simulink model "tracking_model"  (R2017a)
settings: Solver=VariableStepAuto  StartTime=0.0  StopTime=10.0  RelTol=1e-3
values from neighbouring files (symbols this model uses):
  x0 = 100    [validate_model.m]
undefined symbols (not defined in the file or in its folder): sys
(part 14 of 14)

== matlab function tracking_model/Plant/Dynamic system/Mass_block/mass_tensor ==
  data: in1 input; M_matrix output
function M_matrix = Mass_matrix(in1)

%    This function was generated by the Symbolic Math Toolbox version 7.2.

%    10-Jan-2021 16:43:29



th = in1(3,:);

th1 = in1(4,:);

th2 = in1(5,:);

th3 = in1(6,:);

t2 = cos(th);

t3 = cos(th1);

t4 = cos(th2);

t5 = cos(th3);

t6 = sin(th);

t8 = t2.*(1.0./8.0);

t9 = sqrt(3.0);

t10 = t6.*t9.*(1.0./8.0);

t7 = t8-t10;

t11 = t8+t10;

t13 = t6.*(1.0./8.0);

t14 = t2.*t9.*(1.0./8.0);

t12 = t13-t14;

t15 = t13+t14;

M_matrix = reshape([2.11e2./5.0e2,0.0,0.0,0.0,0.0,0.0,0.0,2.11e2./5.0e2,0.0,0.0,0.0,0.0,0.0,0.0,t2.^2.*4.625e-3+t3.^2.*2.518133623269337e-7+t4.^2.*2.518133623269337e-7+t5.^2.*2.518133623269337e-7+t6.^2.*4.625e-3+t7.^2.*(3.7e1./5.0e2)+t11.^2.*(3.7e1./5.0e2)+t12.^2.*(3.7e1./5.0e2)+t15.^2.*(3.7e1./5.0e2)+2.520833333333333e-4,0.0,0.0,0.0,0.0,0.0,0.0,0.0,0.0,0.0,0.0,0.0,0.0,0.0,0.0,0.0,0.0,0.0,0.0,0.0,0.0,0.0],[6,6]);

end

== matlab function tracking_model/Plant/Dynamic system/Auxiliary_matrices/C_matrix ==
  data: in1 input; C output
function C = ConstraintMatrix(in1)

%    This function was generated by the Symbolic Math Toolbox version 7.2.

%    10-Jan-2021 16:43:29



th = in1(3,:);

t2 = pi.*(1.0./3.0);

t3 = t2+th;

C = reshape([1.0,0.0,0.0,sin(th).*(5.0e2./4.3e1),cos(th+pi.*(1.0./6.0)).*(5.0e2./4.3e1),sin(t3).*(-5.0e2./4.3e1),0.0,1.0,0.0,cos(th).*(-5.0e2./4.3e1),cos(th-pi.*(1.0./3.0)).*(5.0e2./4.3e1),cos(t3).*(5.0e2./4.3e1),0.0,0.0,1.0,-1.25e2./4.3e1,-1.25e2./4.3e1,-1.25e2./4.3e1],[6,3]);

end

== matlab function tracking_model/trajectory_function ==
  data: t input; trajs output
function trajs = TrajectoryGenerator(t)

%    This function was generated by the Symbolic Math Toolbox version 7.2.

%    10-Jan-2021 16:30:39



trajs = [cos(t.*1.0e1);sin(t.*1.0e1).*-1.0e1;cos(t.*1.0e1).*-1.0e2;sin(t.*1.0e1);cos(t.*1.0e1).*1.0e1;sin(t.*1.0e1).*-1.0e2;t.*1.0e1;1.0e1;0.0];

end

== matlab function tracking_model/Plant/Dynamic system/Efforts/Constrained_efforts ==
  data: in1 input; fs output; in2 input
function fs = ConstrainedEffort(in1,in2)

%    This function was generated by the Symbolic Math Toolbox version 7.2.

%    10-Jan-2021 16:43:30



p1 = in1(7,:);

p2 = in1(8,:);

p3 = in1(9,:);

tau1 = in2(1,:);

tau2 = in2(2,:);

tau3 = in2(3,:);

th = in1(3,:);

th1 = in1(4,:);

th2 = in1(5,:);

th3 = in1(6,:);

t2 = sin(th);

t3 = sqrt(3.0);

t4 = cos(th);

t5 = p3.^2;

t6 = t2.*t3;

t7 = cos(th2);

t8 = sin(th2);

t9 = th+1.047197551196598;

t10 = cos(th3);

t11 = sin(th3);

t12 = cos(th1);

t13 = sin(th1);

t14 = p3.*t2.*1.25e-1;

t36 = p3.*t4.*2.165063509461097e-1;

t35 = -t36;

t33 = -t35;

t28 = -t33;

t17 = -t28;

t15 = -t17;

t16 = t14+t15;

t18 = t4.*1.25e-1;

t37 = p3.*t4.*-1.25e-1;

t31 = -t37;

t30 = -t31;

t19 = -t30;

t34 = p3.*t2.*2.165063509461097e-1;

t32 = -t34;

t20 = -t32;

t21 = t4.*2.165063509461097e-1;

t22 = p2.*-1.0;

t23 = t19+t20+t22;

t24 = t2.*1.25e-1;

t25 = t21-t24;

t26 = t2.*2.165063509461097e-1;

t27 = t18+t26;

t29 = t21+t24;

t38 = p3.*t4.*(1.0./4.0);

t39 = p2+t38;

t40 = p3.*t2.*-2.5e-1;

t41 = p1+t40;

t42 = th+5.235987755982989e-1;

t43 = cos(t42);

t44 = th-1.047197551196598;

t45 = cos(t44);

t46 = p3.*(1.25e2./4.3e1);

t47 = cos(t9);

t48 = sin(t9);

fs = [t2.*tau1.*(5.0e2./4.3e1)-tau2.*(t2-t3.*t4).*(2.5e2./4.3e1)-tau3.*(t2+t3.*t4).*(2.5e2./4.3e1)-t2.*t5.*t12.*t13.*2.928062352638764e-6-t5.*t7.*t8.*t43.*2.928062352638764e-6+t5.*t10.*t11.*t48.*2.928062352638764e-6;tau2.*(t4+t6).*(2.5e2./4.3e1)-t4.*tau1.*(5.0e2./4.3e1)+tau3.*(t4-t6).*(2.5e2./4.3e1)+t4.*t5.*t12.*t13.*2.928062352638764e-6-t5.*t7.*t8.*t45.*2.928062352638764e-6-t5.*t10.*t11.*t47.*2.928062352638764e-6;tau1.*(-1.25e2./4.3e1)-tau2.*(1.25e2./4.3e1)-tau3.*(1.25e2./4.3e1)-t16.*t23.*(3.7e1./5.0e2)+p3.*(t25.*(t19+t20).*7.4e-2+t2.*t39.*1.85e-2+t16.*t27.*(3.7e1./5.0e2)+t4.*t41.*1.85e-2-t23.*t25.*(3.7e1./5.0e2)+(t14+t17).*(t18-t26).*(3.7e1./5.0e2)-t29.*(t19-p3.*t2.*2.165063509461097e-1).*7.4e-2-t27.*(p1+t14+t28).*7.4e-2-t29.*(p2+t20+t30).*7.4e-2-(t18-t26).*(p1+t14+t17).*7.4e-2).*1.0+(t31+t32).*(p1+t14+t33).*7.4e-2+(t31+t34).*(p1+t14+t35).*7.4e-2+(t14+t36).*(p2+t34+t37).*7.4e-2-p3.*t2.*t39.*1.85e-2-p3.*t4.*t41.*1.85e-2+t5.*t7.*t8.*7.32015588159691e-7+t5.*t10.*t11.*7.32015588159691e-7+t5.*t12.*t13.*7.32015588159691e-7-p3.*t12.*t13.*(t46-p1.*t2.*1.162790697674419e1+p2.*t4.*(5.0e2./4.3e1)).*5.036267246538674e-7-p3.*t10.*t11.*(t46+p1.*t48.*(5.0e2./4.3e1)-p2.*t47.*1.162790697674419e1).*5.036267246538674e-7+p3.*t7.*t8.*(p3.*-2.906976744186047+p1.*t43.*(5.0e2./4.3e1)+p2.*t45.*(5.0e2./4.3e1)).*5.036267246538674e-7];

end

== matlab function tracking_model/Plant/Dynamic system/Mass_block/H ==
  data: C_matrix input; H output; M input
function H = ConstrinedMassMatrix(C_matrix, M)
% MASSMATRIX
%    This function was generated by the Symbolic Math Toolbox version 7.2.
%    16-Oct-2020 11:55:07

    H = C_matrix'*M*C_matrix;
end

== matlab function tracking_model/Plant/Dynamic system/Mass_block/invH ==
  data: matrix input; inv_matrix output
function inv_matrix = matrix_inverse(matrix)
% MASSMATRIX
%    This function was generated by the Symbolic Math Toolbox version 7.2.
%    16-Oct-2020 11:55:07

    inv_matrix = inv(matrix);
end

== matlab function tracking_model/Plant/Dynamic system/Auxiliary_matrices/C_p ==
  data: in1 input; qp output
function qp = KinematicVector(in1)

%    This function was generated by the Symbolic Math Toolbox version 7.2.

%    10-Jan-2021 16:43:29



p1 = in1(7,:);

p2 = in1(8,:);

p3 = in1(9,:);

th = in1(3,:);

t2 = pi.*(1.0./3.0);

t3 = t2+th;

qp = [p1;p2;p3;p3.*(-1.25e2./4.3e1)-p2.*cos(th).*(5.0e2./4.3e1)+p1.*sin(th).*(5.0e2./4.3e1);p3.*(-1.25e2./4.3e1)+p2.*cos(th-pi.*(1.0./3.0)).*(5.0e2./4.3e1)+p1.*cos(th+pi.*(1.0./6.0)).*(5.0e2./4.3e1);p3.*(-1.25e2./4.3e1)+p2.*cos(t3).*(5.0e2./4.3e1)-p1.*sin(t3).*(5.0e2./4.3e1)];

end
